simulink model "demo2"  (R2016a)
settings: Solver=ode45  StartTime=0.0  StopTime=0.1  RelTol=1e-3
values from neighbouring files (symbols this model uses):
  i = i + 1    (= 1)    [demo5.m]
settings Model: Creator=sdudent  LastModifiedBy=Administrator
settings DataIOCC: LimitDataPoints=on  SaveFormat=Array  SignalLoggingSaveFormat=ModelDataLogs
settings OptimizationCC: ExpressionDepthLimit=2147483647
settings DebuggingCC: UnderspecifiedInitializationDetection=Classic  MergeDetectMultiDrivingBlocksExec=none  SolverPrmCheckMsg=warning  FcnCallInpInsideContextMsg=UseLocalSettings  StateNameClashWarn=warning
settings HardwareCC: ProdBitPerPointer=32  ProdLargestAtomicFloat=None  ProdIntDivRoundTo=Undefined  ProdEndianess=Unspecified  ProdWordSize=32  ProdHWDeviceType=32-bit Generic
settings ModelReferenceCC: PropagateSignalLabelsOutOfModel=off
settings GRTTargetCC: CombineOutputUpdateFcns=off  GRTInterface=on
settings ConfigComp: CovModelRefEnable=Off

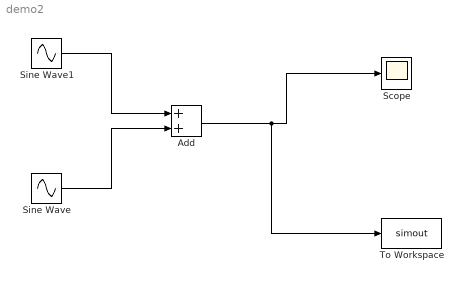
== system demo2 ==
  Add : Sum
  Scope : Scope
  Sine Wave : Sin  Amplitude=i  Frequency=2*pi*150  Phase=30  SampleTime=0
  Sine Wave1 : Sin  Amplitude=100  Frequency=2*pi*50  SampleTime=0
  To Workspace : ToWorkspace  VariableName=simout  SampleTime=-1
  wires:
  Sine Wave1/1 -> Add/1
  Sine Wave/1 -> Add/2
  Add/1 -> Scope/1, To Workspace/1
